simulink model "PVModel3"  (R2023a)
settings: Solver=VariableStepAuto  StartTime=0.0  StopTime=7.4  RelTol=1e-3
values from neighbouring files (symbols this model uses):
  A = 1.3    [PV_Params.mat]    (also in PVparamsforV3.m)
  Isc = 8.61    [PV_Params.mat]    (also in PVparamsforV3.m)
  Ki = 0.05    [PV_Params.mat]    (also in PVparamsforV3.m = 0.0005; paramsv1.m = 0.0017)
  Kv = -0.32    [PV_Params.mat]    (also in PVparamsforV3.m = -0.0032)
  Ns = 60    [PV_Params.mat]    (also in PVparamsforV3.m)
  Rp = 415    [PV_Params.mat]    (also in PVparamsforV3.m)
  Rs = 0.22    [PV_Params.mat]    (also in PVparamsforV3.m)
  Voc = 37.41    [PV_Params.mat]    (also in PVparamsforV3.m)
settings Model: Creator=lucea  LastModifiedBy=lucea

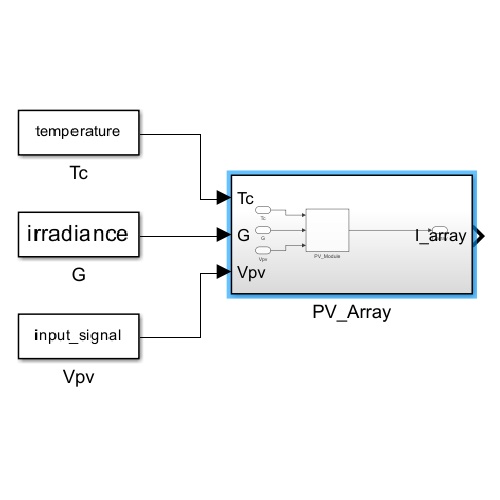
[thumbnail: Simulink's stored preview of the top-level diagram]
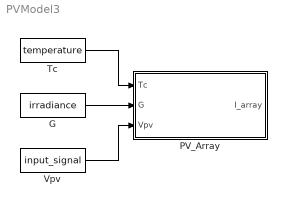
== system PVModel3 ==
  G : FromWorkspace  VariableName=irradiance
  PV_Array : Subsystem
  Tc : FromWorkspace  VariableName=temperature
  Vpv : FromWorkspace  VariableName=input_signal
  wires:
  G/1 -> PV_Array/2(G)
  Tc/1 -> PV_Array/1(Tc)
  Vpv/1 -> PV_Array/3(Vpv)

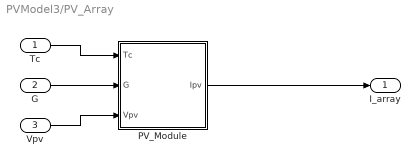
== system PVModel3/PV_Array ==
  Tc : Inport
  G : Inport  Port=2
  Vpv : Inport  Port=3
  PV_Module : Subsystem
  I_array : Outport
  wires:
  PV_Module/1(Ipv) -> I_array/1
  Vpv/1 -> PV_Module/3(Vpv)
  G/1 -> PV_Module/2(G)
  Tc/1 -> PV_Module/1(Tc)

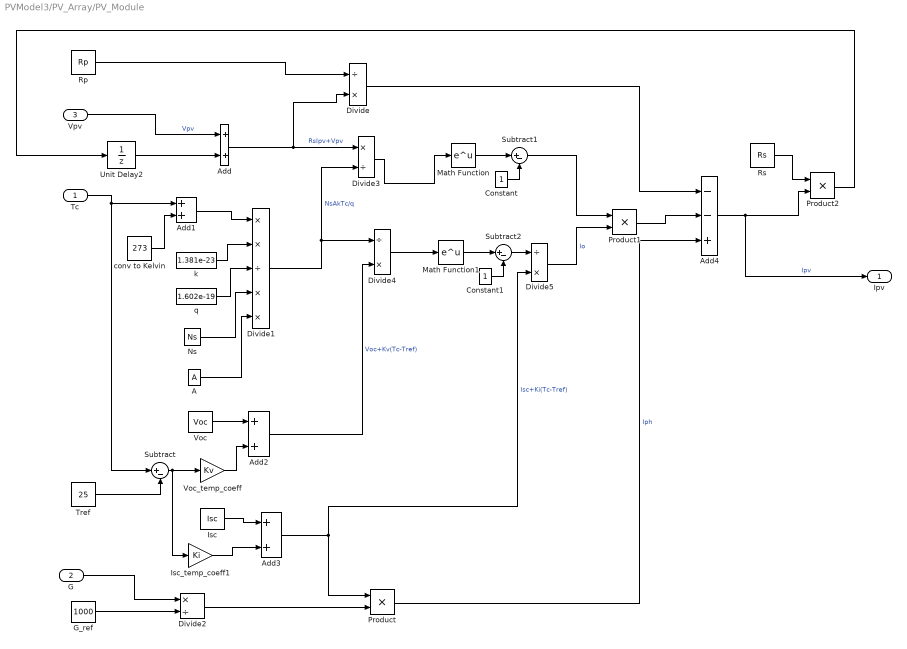
== system PVModel3/PV_Array/PV_Module ==
  Tc : Inport
  G : Inport  Port=2
  Vpv : Inport  Port=3
  A : Constant  Value=A
  Add{,1..3} (4 alike) : Sum
  Add4 : Sum  Inputs=--+
  Constant : Constant
  Constant1 : Constant
  Divide : Product  Inputs=/*
  Divide1 : Product  Inputs=**/**
  Divide2 : Product  Inputs=*/
  Divide3 : Product  Inputs=*/
  Divide4 : Product  Inputs=/*
  Divide5 : Product  Inputs=/*
  G_ref : Constant  Value=1000
  Isc : Constant  Value=Isc
  Isc_temp_coeff1 : Gain  Gain=Ki
  Math Function : Math
  Math Function1 : Math
  Ns : Constant  Value=Ns
  Product : Product
  Product1 : Product
  Product2 : Product
  Rp : Constant  Value=Rp
  Rs : Constant  Value=Rs
  Subtract : Sum  Inputs=|+-
  Subtract1 : Sum  Inputs=|+-
  Subtract2 : Sum  Inputs=|+-
  Tref : Constant  Value=25
  Unit Delay2 : UnitDelay  SampleTime=-1  HasFrameUpgradeWarning=on
  Voc : Constant  Value=Voc
  Voc_temp_coeff : Gain  Gain=Kv
  conv to Kelvin : Constant  Value=273
  k : Constant  Value=1.381e-23
  q : Constant  Value=1.602e-19
  Ipv : Outport
  wires:
  Add1/1 -> Divide1/1
  Product/1 -> Add4/3  "Iph"
  k/1 -> Divide1/2
  Vpv/1 -> Add/1  "Vpv"
  Constant/1 -> Subtract1/2
  Add/1 -> Divide/2, Divide3/1  "RsIpv+Vpv"
  Divide5/1 -> Product1/2  "Io"
  Tc/1 -> Subtract/1, Add1/1
  Add3/1 -> Divide5/2, Product/1  "Isc+Ki(Tc-Tref)"
  Constant1/1 -> Subtract2/2
  Subtract1/1 -> Product1/1
  Divide4/1 -> Math Function1/1
  Divide1/1 -> Divide4/1, Divide3/2  "NsAkTc/q"
  Product1/1 -> Add4/2
  Math Function/1 -> Subtract1/1
  q/1 -> Divide1/3
  Isc/1 -> Add3/1
  Voc_temp_coeff/1 -> Add2/2
  A/1 -> Divide1/5
  Tref/1 -> Subtract/2
  G_ref/1 -> Divide2/2
  Add4/1 -> Product2/2, Ipv/1  "Ipv"
  conv to Kelvin/1 -> Add1/2
  G/1 -> Divide2/1
  Subtract/1 -> Isc_temp_coeff1/1, Voc_temp_coeff/1
  Rp/1 -> Divide/1
  Ns/1 -> Divide1/4
  Isc_temp_coeff1/1 -> Add3/2
  Voc/1 -> Add2/1
  Math Function1/1 -> Subtract2/1
  Add2/1 -> Divide4/2  "Voc+Kv(Tc-Tref)"
  Subtract2/1 -> Divide5/1
  Rs/1 -> Product2/1
  Divide2/1 -> Product/2
  Divide3/1 -> Math Function/1
  Divide/1 -> Add4/1
  Product2/1 -> Unit Delay2/1
  Unit Delay2/1 -> Add/2
